simulink model "UAES_PV"  (R2023b)
settings: Solver=ode45  StartTime=0*24*3600  StopTime=24*3600*365  MaxStep=60  RelTol=1e-4  EnableMultiTasking=on
values from neighbouring files (symbols this model uses):
  P_Inv_W_max = 5100    [PV_code.m]    (also in UAES_ws_PV.mat = 3600)
  sample_time = 3600    [PV_code.m]    (also in Prof_UAEScode.m; UAES_ws_HP.mat; UAES_ws_PV.mat)
undefined symbols (not defined in the file or in its folder): path_carnot, phase
libraries: carnot x4
settings Model: Creator=drhf  LastModifiedBy=Rohan
settings SolverCC: AlgebraicLoopSolver=TrustRegion
settings DataIOCC: LimitDataPoints=on  SaveFormat=Array  ReturnWorkspaceOutputs=off
settings OptimizationCC: ExpressionDepthLimit=2147483647  LifeSpan=inf
settings DebuggingCC: UnderspecifiedInitializationDetection=Classic  MergeDetectMultiDrivingBlocksExec=none  SolverPrmCheckMsg=warning  FcnCallInpInsideContextMsg=warning  UnconnectedInputMsg=warning  UnconnectedOutputMsg=warning  UnconnectedLineMsg=warning  StateNameClashWarn=warning  SFUnexpectedBacktrackingDiag=warning  SFNoUnconditionalDefaultTransitionDiag=warning  SFExecutionAtInitializationDiag=none  ArithmeticOperatorsInVariantConditions=warning
settings HardwareCC: ProdBitPerPointer=32  ProdBitPerSizeT=32  ProdBitPerPtrDiffT=32  ProdLargestAtomicFloat=None  ProdIntDivRoundTo=Undefined  ProdEndianess=Unspecified  ProdWordSize=32  ProdHWDeviceType=32-bit Generic
settings ModelReferenceCC: EnableRefExpFcnMdlSchedulingChecks=on  PropagateSignalLabelsOutOfModel=off
settings SFSimCC: SimUseLocalCustomCode=off  CustomCodeUndefinedFunction=UseInterfaceOnly
settings RTWCC: RTWUseLocalCustomCode=off
settings CodeAppCC: StateflowObjectComments=on
settings GRTTargetCC: TargetLangStandard=C89/C90 (ANSI)  CombineOutputUpdateFcns=off  GRTInterface=on
settings ConfigComp: CovMetricSettings=dw  CovSaveCumulativeToWorkspaceVar=on  CovSaveSingleToWorkspaceVar=on  CovExternalEMLEnable=off

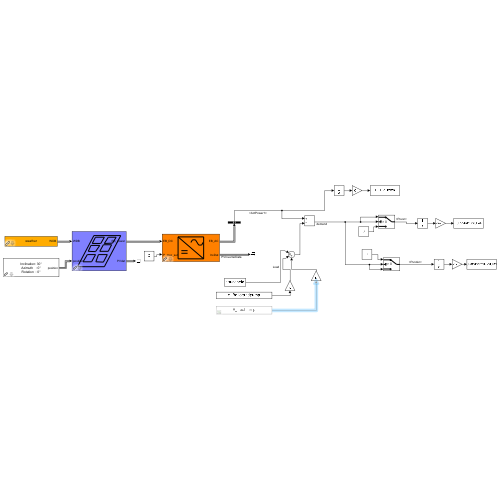
[thumbnail: Simulink's stored preview of the top-level diagram]
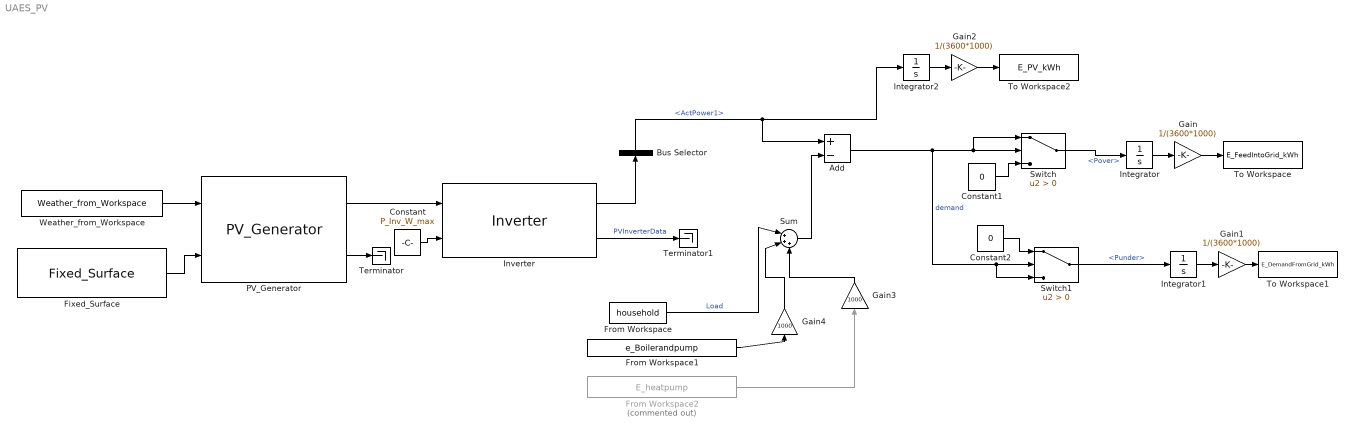
== system UAES_PV ==
  Add : Sum  Inputs=+-
  Bus Selector : BusSelector  OutputSignals=ActPower1
  Constant : Constant  Value=P_Inv_W_max
  Constant1 : Constant  Value=0
  Constant2 : Constant  Value=0
  Fixed_Surface : carnot/Weather/Fixed_Surface  colangle=30  colazi=0  colrot=0
  From Workspace : FromWorkspace  VariableName=household  OutputAfterFinalValue=Setting to zero
  From Workspace1 : FromWorkspace  VariableName=e_Boilerandpump
  From Workspace2 : FromWorkspace  Commented=on  VariableName=E_heatpump
  Gain : Gain  Gain=1/(3600*1000)
  Gain1 : Gain  Gain=1/(3600*1000)
  Gain2 : Gain  Gain=1/(3600*1000)
  Gain3 : Gain  Gain=1000
  Gain4 : Gain  Gain=1000
  Integrator : Integrator
  Integrator1 : Integrator
  Integrator2 : Integrator
  Inverter : carnot/Source/Electric_Generator/Inverter  PathName=fullfile(path_carnot('libsl'), 'Source','Electric_Generator','Inverter','parameter_set')  FileName='<user defined>'  userPath=off  userParam=on  Pacnom=P_Inv_W  nphase=1-phase  U=230  f=50  PstepsEta=[0 0.1 0.2 0.25 0.3 0.5 0.75 1]  Eta=[0 0.948 0.966 0.969 0.97 0.972 0.97 0.967]  P_standby=2
  PV_Generator : carnot/Source/Electric_Generator/PV_Generator  Wp=PV_W  delta_Wp_K=0.0047  fgen=0.91 % 0.06 power missmatch, 0.01 diodes, 0.02 data sheet tolerance
  Sum : Sum  Inputs=|+++
  Switch : Switch  Criteria=u2 > Threshold  SaturateOnIntegerOverflow=off  InputSameDT=off
  Switch1 : Switch  Criteria=u2 > Threshold  SaturateOnIntegerOverflow=off  InputSameDT=off
  Terminator : Terminator
  Terminator1 : Terminator
  To Workspace : ToWorkspace  VariableName=E_FeedIntoGrid_kWh  SampleTime=sample_time
  To Workspace1 : ToWorkspace  VariableName=E_DemandFromGrid_kWh  SampleTime=sample_time
  To Workspace2 : ToWorkspace  VariableName=E_PV_kWh  SampleTime=sample_time
  Weather_from_Workspace : carnot/Weather/Weather_from_Workspace  file=weather
  wires:
  PV_Generator/1 -> Inverter/1
  Fixed_Surface/1 -> PV_Generator/2
  Weather_from_Workspace/1 -> PV_Generator/1
  PV_Generator/2 -> Terminator/1
  Constant/1 -> Inverter/2
  Inverter/2 -> Terminator1/1  "PVInverterData"
  Bus Selector/1 -> Add/1, Integrator2/1  "<ActPower1>"
  Add/1 -> Switch1/3, Switch1/2, Switch/1, Switch/2  "demand"
  Inverter/1 -> Bus Selector/1
  From Workspace/1 -> Sum/1  "Load"
  Integrator2/1 -> Gain2/1
  Gain2/1 -> To Workspace2/1
  Integrator/1 -> Gain/1
  Switch/1 -> Integrator/1  "<Pover>"
  Gain/1 -> To Workspace/1
  Integrator1/1 -> Gain1/1
  Gain1/1 -> To Workspace1/1
  Switch1/1 -> Integrator1/1  "<Punder>"
  Constant1/1 -> Switch/3
  Constant2/1 -> Switch1/1
  From Workspace1/1 -> Gain4/1
  From Workspace2/1 -> Gain3/1
  Sum/1 -> Add/2
  Gain4/1 -> Sum/2
  Gain3/1 -> Sum/3
